simulink model "Robotic_Arm_For_SIMScape_2"  (R2020a)
settings: Solver=FixedStepAuto  StartTime=0.0  StopTime=70  FixedStep=0.01  RelTol=1e-3
model workspace: external: MATLAB File D:\jsp\Nottingham\Year 4\Semester 2\Third Year Project - Autonomous Robotic Arm\Software Development\SimScape\Version2\Robotic_Arm_For_SIMScape_2_DataFile.m (data not in the file)
values from neighbouring files (symbols this model uses):
  fcn11 = VariableA1(1)    [MainCode_16522575.m]
  fcn12 = VariableA1(2)    [MainCode_16522575.m]
  fcn13 = VariableA1(3)    [MainCode_16522575.m]
  fcn14 = VariableA1(4)    [MainCode_16522575.m]
  fcn1_1place = VariableA1toPlace(1)    [MainCode_16522575.m]
  fcn1_1placetoPrevious = VariableA1toPlacetoPrevious(1)    [MainCode_16522575.m]
  fcn1_2place = VariableA1toPlace(2)    [MainCode_16522575.m]
  fcn1_2placetoPrevious = VariableA1toPlacetoPrevious(2)    [MainCode_16522575.m]
  fcn1_3place = VariableA1toPlace(3)    [MainCode_16522575.m]
  fcn1_3placetoPrevious = VariableA1toPlacetoPrevious(3)    [MainCode_16522575.m]
  fcn1_4place = VariableA1toPlace(4)    [MainCode_16522575.m]
  fcn1_4placetoPrevious = VariableA1toPlacetoPrevious(4)    [MainCode_16522575.m]
  fcn21 = VariableA2(1)    [MainCode_16522575.m]
  fcn21home = VariableA2home(1)    [MainCode_16522575.m]
  fcn22 = VariableA2(2)    [MainCode_16522575.m]
  fcn22home = VariableA2home(2)    [MainCode_16522575.m]
  fcn23 = VariableA2(3)    [MainCode_16522575.m]
  fcn23home = VariableA2home(3)    [MainCode_16522575.m]
  fcn24 = VariableA2(4)    [MainCode_16522575.m]
  fcn24home = VariableA2home(4)    [MainCode_16522575.m]
  fcn2_1place = VariableA2toPlace(1)    [MainCode_16522575.m]
  fcn2_1placetohome = VariableA2toPlacetohome(1)    [MainCode_16522575.m]
  fcn2_2place = VariableA2toPlace(2)    [MainCode_16522575.m]
  fcn2_2placetohome = VariableA2toPlacetohome(2)    [MainCode_16522575.m]
  fcn2_3place = VariableA2toPlace(3)    [MainCode_16522575.m]
  fcn2_3placetohome = VariableA2toPlacetohome(3)    [MainCode_16522575.m]
  fcn2_4place = VariableA2toPlace(4)    [MainCode_16522575.m]
  fcn2_4placetohome = VariableA2toPlacetohome(4)    [MainCode_16522575.m]
  fcn31 = VariableA3(1)    [MainCode_16522575.m]
  fcn31home = VariableA3home(1)    [MainCode_16522575.m]
  fcn32 = VariableA3(2)    [MainCode_16522575.m]
  fcn32home = VariableA3home(2)    [MainCode_16522575.m]
  fcn33 = VariableA3(3)    [MainCode_16522575.m]
  fcn33home = VariableA3home(3)    [MainCode_16522575.m]
  fcn34 = VariableA3(4)    [MainCode_16522575.m]
  fcn34home = VariableA3home(4)    [MainCode_16522575.m]
  fcn3_1place = VariableA3toPlace(1)    [MainCode_16522575.m]
  fcn3_1placetohome = VariableA3toPlacetohome(1)    [MainCode_16522575.m]
  fcn3_2place = VariableA3toPlace(2)    [MainCode_16522575.m]
  fcn3_2placetohome = VariableA3toPlacetohome(2)    [MainCode_16522575.m]
  fcn3_3place = VariableA3toPlace(3)    [MainCode_16522575.m]
  fcn3_3placetohome = VariableA3toPlacetohome(3)    [MainCode_16522575.m]
  fcn3_4place = VariableA3toPlace(4)    [MainCode_16522575.m]
  fcn3_4placetohome = VariableA3toPlacetohome(4)    [MainCode_16522575.m]
  qd1_final = qd1(1000)    [TrajectoryPlanning.m]
  qd1_finalplace = qd1toPlace(1000)    [TrajectoryPlanning1toPlace.m]
  qd2_finalhome = qd2home(1000)    [TrajectoryPlanning2tohome.m]
  qd2_finalplacetohome = qd2toPlacetohome(1000)    [TrajectoryPlanning2Placetohome.m]
  qd2_initial = qd2(1)    [TrajectoryPlanning2.m]
  qd3_finalhome = qd3home(1000)    [TrajectoryPlanning3tohome.m]
  qd3_finalplacetohome = qd3toPlacetohome(1000)    [TrajectoryPlanning3Placetohome.m]
  qd3_initial = qd3(1)    [TrajectoryPlanning3.m]
  s = z-d1    [InverseKinematics.m]
undefined symbols (not defined in the file or in its folder): sigbuilder_block, smiData, X, Y, Z
libraries: sm_lib x32, nesl_utility x15
(part 1 of 2)
settings Model: Creator=sp_ja  LastModifiedBy=sp_ja
settings OptimizationCC: BlockReduction=off  DefaultParameterBehavior=Inlined  BufferReuse=off

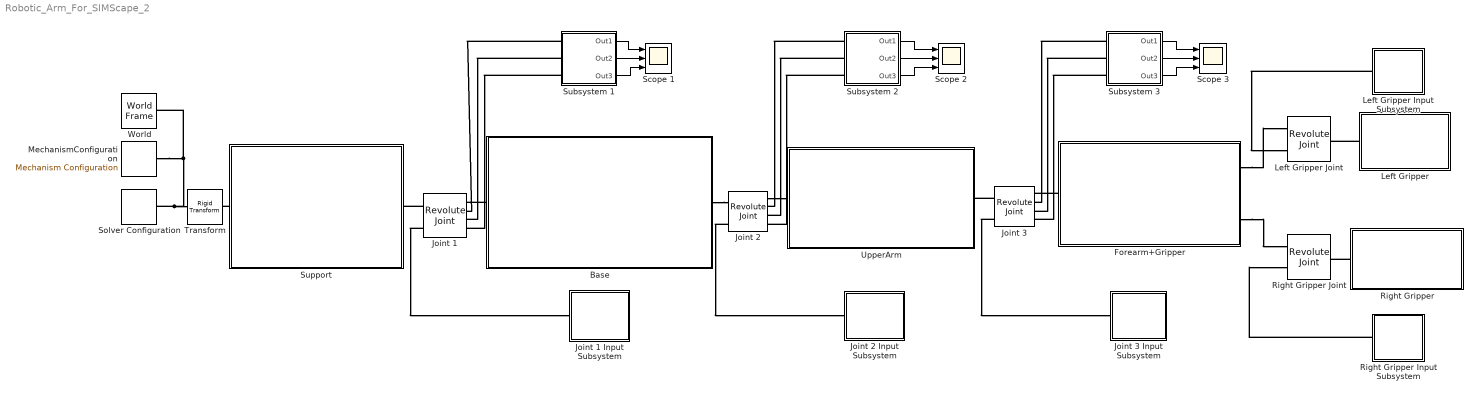
== system Robotic_Arm_For_SIMScape_2 ==
  Base : Subsystem
      mask Display: image('D:\jsp\Nottingham\Year 4\Semester 2\Third Year Project - Autonomous Robotic Arm\Software Development\SimScape\Version2\Pictures for Simulink\BaseNew.JPG'); % Use "Edit Image" on toolstrip to change.
  Forearm+Gripper : Subsystem
      mask Display: image('D:\jsp\Nottingham\Year 4\Semester 2\Third Year Project - Autonomous Robotic Arm\Software Development\SimScape\Version2\Pictures for Simulink\UpperArmNew3.JPG'); % Use "Edit Image" on toolstrip to change.
  "Joint 1 " : sm_lib/Joints/Revolute Joint  JointMode=Normal  SenseConstraintForce=off  SenseConstraintForceX=off  SenseConstraintForceY=off  SenseConstraintForceZ=off  SenseConstraintTorque=off  SenseConstraintTorqueX=off  SenseConstraintTorqueY=off  SenseConstraintTorqueZ=off  SenseTotalForce=off  SenseTotalForceX=off  SenseTotalForceY=off  SenseTotalForceZ=off  SenseTotalTorque=off  SenseTotalTorqueX=off  SenseTotalTorqueY=off  SenseTotalTorqueZ=off  CompositeWrenchDir=FollowerOnBase  CompositeWrenchFrame=BaseFrame  EquilibriumPosition=0  EquilibriumPositionUnits=rad  SpringStiffness=0  SpringStiffnessUnits=N*m/rad  DampingCoefficient=0  DampingCoefficientUnits=N*m/(rad/s)  TorqueActuationMode=ComputedTorque  MotionActuationMode=InputMotion  SensePosition=on  SenseVelocity=on  SenseAcceleration=on  SenseTorqueForce=off  SenseLowerLimitTorqueForce=off  SenseUpperLimitTorqueForce=off  LowerLimitSpecify=off  LowerLimitBound=-90  LowerLimitBoundUnits=deg  LowerLimitStiffness=1e4  LowerLimitStiffnessUnits=N*m/deg  LowerLimitDamping=10  LowerLimitDampingUnits=N*m/(deg/s)  LowerLimitTransitionRegionWidth=0.1  LowerLimitTransitionRegionWidthUnits=deg  UpperLimitSpecify=off  UpperLimitBound=90  UpperLimitBoundUnits=deg  UpperLimitStiffness=1e4  UpperLimitStiffnessUnits=N*m/deg  UpperLimitDamping=10  UpperLimitDampingUnits=N*m/(deg/s)  UpperLimitTransitionRegionWidth=0.1  UpperLimitTransitionRegionWidthUnits=deg  PositionTargetSpecify=on  PositionTargetPriority=Low  PositionTargetValue=smiData.RevoluteJoint(2).Rz.Pos  PositionTargetValueUnits=deg  VelocityTargetSpecify=off  VelocityTargetPriority=High  VelocityTargetValue=0  VelocityTargetValueUnits=deg/s
  Joint 1 Input Subsystem : Subsystem
      mask Display: image('D:\jsp\Nottingham\Year 4\Semester 2\Third Year Project - Autonomous Robotic Arm\Software Development\SimScape\Version2\Pictures for Simulink\return.png'); % Use "Edit Image" on toolstrip to change.
  Joint 2 : sm_lib/Joints/Revolute Joint  JointMode=Normal  SenseConstraintForce=off  SenseConstraintForceX=off  SenseConstraintForceY=off  SenseConstraintForceZ=off  SenseConstraintTorque=off  SenseConstraintTorqueX=off  SenseConstraintTorqueY=off  SenseConstraintTorqueZ=off  SenseTotalForce=off  SenseTotalForceX=off  SenseTotalForceY=off  SenseTotalForceZ=off  SenseTotalTorque=off  SenseTotalTorqueX=off  SenseTotalTorqueY=off  SenseTotalTorqueZ=off  CompositeWrenchDir=FollowerOnBase  CompositeWrenchFrame=BaseFrame  EquilibriumPosition=0  EquilibriumPositionUnits=rad  SpringStiffness=0  SpringStiffnessUnits=N*m/rad  DampingCoefficient=0  DampingCoefficientUnits=N*m/(rad/s)  TorqueActuationMode=ComputedTorque  MotionActuationMode=InputMotion  SensePosition=on  SenseVelocity=on  SenseAcceleration=on  SenseTorqueForce=off  SenseLowerLimitTorqueForce=off  SenseUpperLimitTorqueForce=off  LowerLimitSpecify=off  LowerLimitBound=-90  LowerLimitBoundUnits=deg  LowerLimitStiffness=1e4  LowerLimitStiffnessUnits=N*m/deg  LowerLimitDamping=10  LowerLimitDampingUnits=N*m/(deg/s)  LowerLimitTransitionRegionWidth=0.1  LowerLimitTransitionRegionWidthUnits=deg  UpperLimitSpecify=off  UpperLimitBound=90  UpperLimitBoundUnits=deg  UpperLimitStiffness=1e4  UpperLimitStiffnessUnits=N*m/deg  UpperLimitDamping=10  UpperLimitDampingUnits=N*m/(deg/s)  UpperLimitTransitionRegionWidth=0.1  UpperLimitTransitionRegionWidthUnits=deg  PositionTargetSpecify=on  PositionTargetPriority=Low  PositionTargetValue=smiData.RevoluteJoint(3).Rz.Pos  PositionTargetValueUnits=deg  VelocityTargetSpecify=off  VelocityTargetPriority=High  VelocityTargetValue=0  VelocityTargetValueUnits=deg/s
  Joint 2 Input Subsystem : Subsystem
      mask Display: image('D:\jsp\Nottingham\Year 4\Semester 2\Third Year Project - Autonomous Robotic Arm\Software Development\SimScape\Version2\Pictures for Simulink\return.png'); % Use "Edit Image" on toolstrip to change.
  Joint 3 : sm_lib/Joints/Revolute Joint  JointMode=Normal  SenseConstraintForce=off  SenseConstraintForceX=off  SenseConstraintForceY=off  SenseConstraintForceZ=off  SenseConstraintTorque=off  SenseConstraintTorqueX=off  SenseConstraintTorqueY=off  SenseConstraintTorqueZ=off  SenseTotalForce=off  SenseTotalForceX=off  SenseTotalForceY=off  SenseTotalForceZ=off  SenseTotalTorque=off  SenseTotalTorqueX=off  SenseTotalTorqueY=off  SenseTotalTorqueZ=off  CompositeWrenchDir=FollowerOnBase  CompositeWrenchFrame=BaseFrame  EquilibriumPosition=0  EquilibriumPositionUnits=rad  SpringStiffness=0  SpringStiffnessUnits=N*m/rad  DampingCoefficient=0  DampingCoefficientUnits=N*m/(rad/s)  TorqueActuationMode=ComputedTorque  MotionActuationMode=InputMotion  SensePosition=on  SenseVelocity=on  SenseAcceleration=on  SenseTorqueForce=off  SenseLowerLimitTorqueForce=off  SenseUpperLimitTorqueForce=off  LowerLimitSpecify=off  LowerLimitBound=-90  LowerLimitBoundUnits=deg  LowerLimitStiffness=1e4  LowerLimitStiffnessUnits=N*m/deg  LowerLimitDamping=10  LowerLimitDampingUnits=N*m/(deg/s)  LowerLimitTransitionRegionWidth=0.1  LowerLimitTransitionRegionWidthUnits=deg  UpperLimitSpecify=off  UpperLimitBound=90  UpperLimitBoundUnits=deg  UpperLimitStiffness=1e4  UpperLimitStiffnessUnits=N*m/deg  UpperLimitDamping=10  UpperLimitDampingUnits=N*m/(deg/s)  UpperLimitTransitionRegionWidth=0.1  UpperLimitTransitionRegionWidthUnits=deg  PositionTargetSpecify=on  PositionTargetPriority=Low  PositionTargetValue=smiData.RevoluteJoint(5).Rz.Pos  PositionTargetValueUnits=deg  VelocityTargetSpecify=off  VelocityTargetPriority=High  VelocityTargetValue=0  VelocityTargetValueUnits=deg/s
  Joint 3 Input Subsystem : Subsystem
      mask Display: image('D:\jsp\Nottingham\Year 4\Semester 2\Third Year Project - Autonomous Robotic Arm\Software Development\SimScape\Version2\Pictures for Simulink\return.png'); % Use "Edit Image" on toolstrip to change.
  Left Gripper : Subsystem
      mask Display: image('D:\jsp\Nottingham\Year 4\Semester 2\Third Year Project - Autonomous Robotic Arm\Software Development\SimScape\Version2\Pictures for Simulink\Gripper.JPG'); % Use "Edit Image" on toolstrip to change.
  Left Gripper Input Subsystem : Subsystem
      mask Display: image('D:\jsp\Nottingham\Year 4\Semester 2\Third Year Project - Autonomous Robotic Arm\Software Development\SimScape\Version2\Pictures for Simulink\return.png'); % Use "Edit Image" on toolstrip to change.
  Left Gripper Joint : sm_lib/Joints/Revolute Joint  JointMode=Normal  SenseConstraintForce=off  SenseConstraintForceX=off  SenseConstraintForceY=off  SenseConstraintForceZ=off  SenseConstraintTorque=off  SenseConstraintTorqueX=off  SenseConstraintTorqueY=off  SenseConstraintTorqueZ=off  SenseTotalForce=off  SenseTotalForceX=off  SenseTotalForceY=off  SenseTotalForceZ=off  SenseTotalTorque=off  SenseTotalTorqueX=off  SenseTotalTorqueY=off  SenseTotalTorqueZ=off  CompositeWrenchDir=FollowerOnBase  CompositeWrenchFrame=BaseFrame  EquilibriumPosition=0  EquilibriumPositionUnits=rad  SpringStiffness=0  SpringStiffnessUnits=N*m/rad  DampingCoefficient=0  DampingCoefficientUnits=N*m/(rad/s)  TorqueActuationMode=ComputedTorque  MotionActuationMode=InputMotion  SensePosition=off  SenseVelocity=off  SenseAcceleration=off  SenseTorqueForce=off  SenseLowerLimitTorqueForce=off  SenseUpperLimitTorqueForce=off  LowerLimitSpecify=off  LowerLimitBound=-90  LowerLimitBoundUnits=deg  LowerLimitStiffness=1e4  LowerLimitStiffnessUnits=N*m/deg  LowerLimitDamping=10  LowerLimitDampingUnits=N*m/(deg/s)  LowerLimitTransitionRegionWidth=0.1  LowerLimitTransitionRegionWidthUnits=deg  UpperLimitSpecify=off  UpperLimitBound=90  UpperLimitBoundUnits=deg  UpperLimitStiffness=1e4  UpperLimitStiffnessUnits=N*m/deg  UpperLimitDamping=10  UpperLimitDampingUnits=N*m/(deg/s)  UpperLimitTransitionRegionWidth=0.1  UpperLimitTransitionRegionWidthUnits=deg  PositionTargetSpecify=on  PositionTargetPriority=Low  PositionTargetValue=smiData.RevoluteJoint(4).Rz.Pos  PositionTargetValueUnits=deg  VelocityTargetSpecify=off  VelocityTargetPriority=High  VelocityTargetValue=0  VelocityTargetValueUnits=deg/s
  MechanismConfiguration : sm_lib/Utilities/Mechanism Configuration  UniformGravity=Constant  GravityVector=[0 -9.80665 0]  GravityUnits=m/s^2  LinearizationDelta=0.001
  Right Gripper : Subsystem
      mask Display: image('D:\jsp\Nottingham\Year 4\Semester 2\Third Year Project - Autonomous Robotic Arm\Software Development\SimScape\Version2\Pictures for Simulink\Gripper_with_Trigger.JPG'); % Use "Edit Image" on toolstrip to change.
  Right Gripper Input Subsystem : Subsystem
      mask Display: image('D:\jsp\Nottingham\Year 4\Semester 2\Third Year Project - Autonomous Robotic Arm\Software Development\SimScape\Version2\Pictures for Simulink\return.png'); % Use "Edit Image" on toolstrip to change.
  Right Gripper Joint : sm_lib/Joints/Revolute Joint  JointMode=Normal  SenseConstraintForce=off  SenseConstraintForceX=off  SenseConstraintForceY=off  SenseConstraintForceZ=off  SenseConstraintTorque=off  SenseConstraintTorqueX=off  SenseConstraintTorqueY=off  SenseConstraintTorqueZ=off  SenseTotalForce=off  SenseTotalForceX=off  SenseTotalForceY=off  SenseTotalForceZ=off  SenseTotalTorque=off  SenseTotalTorqueX=off  SenseTotalTorqueY=off  SenseTotalTorqueZ=off  CompositeWrenchDir=FollowerOnBase  CompositeWrenchFrame=BaseFrame  EquilibriumPosition=0  EquilibriumPositionUnits=rad  SpringStiffness=0  SpringStiffnessUnits=N*m/rad  DampingCoefficient=0  DampingCoefficientUnits=N*m/(rad/s)  TorqueActuationMode=ComputedTorque  MotionActuationMode=InputMotion  SensePosition=off  SenseVelocity=off  SenseAcceleration=off  SenseTorqueForce=off  SenseLowerLimitTorqueForce=off  SenseUpperLimitTorqueForce=off  LowerLimitSpecify=off  LowerLimitBound=-90  LowerLimitBoundUnits=deg  LowerLimitStiffness=1e4  LowerLimitStiffnessUnits=N*m/deg  LowerLimitDamping=10  LowerLimitDampingUnits=N*m/(deg/s)  LowerLimitTransitionRegionWidth=0.1  LowerLimitTransitionRegionWidthUnits=deg  UpperLimitSpecify=off  UpperLimitBound=90  UpperLimitBoundUnits=deg  UpperLimitStiffness=1e4  UpperLimitStiffnessUnits=N*m/deg  UpperLimitDamping=10  UpperLimitDampingUnits=N*m/(deg/s)  UpperLimitTransitionRegionWidth=0.1  UpperLimitTransitionRegionWidthUnits=deg  PositionTargetSpecify=on  PositionTargetPriority=Low  PositionTargetValue=smiData.RevoluteJoint(1).Rz.Pos  PositionTargetValueUnits=deg  VelocityTargetSpecify=off  VelocityTargetPriority=High  VelocityTargetValue=0  VelocityTargetValueUnits=deg/s
  Scope 1 : Scope  NumInputPorts=3
  Scope 2 : Scope  NumInputPorts=3
  Scope 3 : Scope  NumInputPorts=3
  Solver Configuration : nesl_utility/Solver Configuration  PhysicalDomain=network_engine_domain  SubClassName=solver  LeftPortType=input  RightPortType=generic  Tones=[]  Harmonics=[]  SimulateNoise=off  Profile=off  UseLocalSampling=off  EnableSwitchedLinearOptims=on  FrequencyDomain=off  UseCCode=off  RelTol=0.001  AbsTol=1e-06  MinStep=1e-09  ToWorkspace=off  RevertToSquareIcSolve=off  NumHomotopyIterations=100  PhasorMode=off  PhasorModeNumHarmonics=1  DoDC=off  ResidualTolerance=1e-09  UseLocalSolver=off  LocalSolverChoice=NE_BACKWARD_EULER_ADVANCER  LocalSolverSampleTime=0.001  DoFixedCost=off  MaxNonlinIter=3  MaxModeIter=2  LinearAlgebra=auto  EquationFormulation=NE_TIME_EF  DelaysMemoryBudget=1024  AutomaticFiltering=on  FilteringTimeConstant=0.001  PartitionStorageMethod=AS_NEEDED  PartitionMemoryBudget=1024  PartitionMethod=ROBUST
  Subsystem 1 : Subsystem
      mask Display: image('D:\jsp\Nottingham\Year 4\Semester 2\Third Year Project - Autonomous Robotic Arm\Software Development\SimScape\Version2\Pictures for Simulink\point-to.png'); % Use "Edit Image" on toolstrip to change.
  Subsystem 2 : Subsystem
      mask Display: image('D:\jsp\Nottingham\Year 4\Semester 2\Third Year Project - Autonomous Robotic Arm\Software Development\SimScape\Version2\Pictures for Simulink\point-to.png'); % Use "Edit Image" on toolstrip to change.
  Subsystem 3 : Subsystem
      mask Display: image('D:\jsp\Nottingham\Year 4\Semester 2\Third Year Project - Autonomous Robotic Arm\Software Development\SimScape\Version2\Pictures for Simulink\point-to.png'); % Use "Edit Image" on toolstrip to change.
  Support : Subsystem
      mask Display: image('D:\jsp\Nottingham\Year 4\Semester 2\Third Year Project - Autonomous Robotic Arm\Software Development\SimScape\Version2\Pictures for Simulink\SupportNew.JPG'); % Use "Edit Image" on toolstrip to change.
  Transform : sm_lib/Frames and Transforms/Rigid Transform  TranslationMethod=Cartesian  TranslationStandardOffset=0  TranslationLengthUnit=mm  TranslationStandardAxis=+Z  TranslationCartesianOffset=smiData.RigidTransform(12).translation  TranslationROffset=0  TranslationROffsetUnits=m  TranslationZOffset=0  TranslationZOffsetUnits=m  TranslationThetaOffset=0  TranslationThetaOffsetUnits=deg  RotationMethod=ArbitraryAxis  RotationAngleUnits=rad  RotationStandardAxis=+Z  RotationAngle=smiData.RigidTransform(12).angle  RotationArbitraryAxis=smiData.RigidTransform(12).axis  FollAlignAxisA=+X  BaseAlignAxisA=+Y  FollAlignAxisB=+Y  BaseAlignAxisB=+Z  RotationSequenceAxes=FollowerAxes  RotationSequence=XYX  RotationSequenceAngles=[0 0 0]  RotationSequenceAnglesUnits=deg  RotationMatrix=[1 0 0; 0 1 0; 0 0 1]
  UpperArm : Subsystem
      mask Display: image('D:\jsp\Nottingham\Year 4\Semester 2\Third Year Project - Autonomous Robotic Arm\Software Development\SimScape\Version2\Pictures for Simulink\Forearm + Gripper without offset.JPG'); % Use "Edit Image" on toolstrip to change.
  World : sm_lib/Frames and Transforms/World Frame
  wires:
  Subsystem 1/1(Out1) -> Scope 1/1
  Subsystem 1/2(Out2) -> Scope 1/2
  Subsystem 1/3(Out3) -> Scope 1/3
  Subsystem 2/1(Out1) -> Scope 2/1
  Subsystem 2/2(Out2) -> Scope 2/2
  Subsystem 2/3(Out3) -> Scope 2/3
  Subsystem 3/1(Out1) -> Scope 3/1
  Subsystem 3/2(Out2) -> Scope 3/2
  Subsystem 3/3(Out3) -> Scope 3/3
  connections:
  MechanismConfiguration/RConn1 -- Solver Configuration/RConn1 -- Transform/LConn1 -- World/RConn1
  Forearm+Gripper/RConn2 -- Right Gripper Joint/LConn1
  Forearm+Gripper/LConn1 -- Joint 3/RConn1
  Support/LConn1 -- Transform/RConn1
  Right Gripper/LConn1 -- Right Gripper Joint/RConn1
  "Joint 1 "/LConn1 -- Support/RConn1
  Base/LConn1 -- "Joint 1 "/RConn1
  Base/RConn1 -- Joint 2/LConn1
  Joint 2/RConn1 -- UpperArm/LConn1
  Forearm+Gripper/RConn1 -- Left Gripper Joint/LConn1
  Left Gripper/LConn1 -- Left Gripper Joint/RConn1
  Joint 3/LConn1 -- UpperArm/RConn1
  Subsystem 1/LConn1 -- "Joint 1 "/RConn2
  Subsystem 1/LConn2 -- "Joint 1 "/RConn3
  Subsystem 1/LConn3 -- "Joint 1 "/RConn4
  Subsystem 2/LConn1 -- Joint 2/RConn2
  Subsystem 2/LConn2 -- Joint 2/RConn3
  Subsystem 2/LConn3 -- Joint 2/RConn4
  Subsystem 3/LConn1 -- Joint 3/RConn2
  Subsystem 3/LConn2 -- Joint 3/RConn3
  Subsystem 3/LConn3 -- Joint 3/RConn4
  "Joint 1 "/LConn2 -- Joint 1 Input Subsystem/RConn1
  Joint 2/LConn2 -- Joint 2 Input Subsystem/RConn1
  Joint 3/LConn2 -- Joint 3 Input Subsystem/RConn1
  Right Gripper Input Subsystem/RConn1 -- Right Gripper Joint/LConn2
  Left Gripper Input Subsystem/RConn1 -- Left Gripper Joint/LConn2

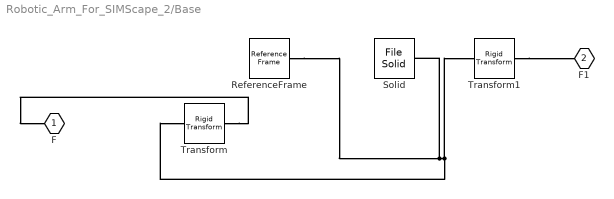
== system Robotic_Arm_For_SIMScape_2/Base ==
  ReferenceFrame : sm_lib/Frames and Transforms/Reference Frame
  Solid : sm_lib/Body Elements/File Solid  ExtGeomFileName=BaseNew_Default_sldprt.STEP  UnitType=FromFile  ExtGeomFileUnits=m  StepReaderType=HEX  ExportConvexHullGeometry=off  InertiaType=Custom  Mass=smiData.Solid(1).mass  MassUnits=kg  CenterOfMass=smiData.Solid(1).CoM  CenterOfMassUnits=mm  MomentsOfInertia=smiData.Solid(1).MoI  MomentsOfInertiaUnits=kg*mm^2  ProductsOfInertia=smiData.Solid(1).PoI  ProductsOfInertiaUnits=kg*mm^2  BasedOnType=DensityFromFile  Density=1000  DensityUnits=kg/m^3  DoExposeReferenceFrame=on  SerializedFrames=<Frames/>  GraphicType=FromGeometry  MarkerShape=Sphere  MarkerSize=10  GraphicVisPropType=AdvancedVisualProperties  GraphicDiffuseColor=[0.0 0.40392157 1.0]  GraphicSpecularColor=[0.5 0.5 0.5 1.0]  GraphicAmbientColor=[0.15 0.15 0.15 1.0]  GraphicEmissiveColor=[0.0 0.0 0.0 1.0]  GraphicShininess=10  GraphicOpacity=smiData.Solid(1).opacity
  Transform : sm_lib/Frames and Transforms/Rigid Transform  TranslationMethod=Cartesian  TranslationStandardOffset=0  TranslationLengthUnit=mm  TranslationStandardAxis=+Z  TranslationCartesianOffset=smiData.RigidTransform(4).translation  TranslationROffset=0  TranslationROffsetUnits=m  TranslationZOffset=0  TranslationZOffsetUnits=m  TranslationThetaOffset=0  TranslationThetaOffsetUnits=deg  RotationMethod=ArbitraryAxis  RotationAngleUnits=rad  RotationStandardAxis=+Z  RotationAngle=smiData.RigidTransform(4).angle  RotationArbitraryAxis=smiData.RigidTransform(4).axis  FollAlignAxisA=+X  BaseAlignAxisA=+Y  FollAlignAxisB=+Y  BaseAlignAxisB=+Z  RotationSequenceAxes=FollowerAxes  RotationSequence=XYX  RotationSequenceAngles=[0 0 0]  RotationSequenceAnglesUnits=deg  RotationMatrix=[1 0 0; 0 1 0; 0 0 1]
  Transform1 : sm_lib/Frames and Transforms/Rigid Transform  TranslationMethod=Cartesian  TranslationStandardOffset=0  TranslationLengthUnit=mm  TranslationStandardAxis=+Z  TranslationCartesianOffset=smiData.RigidTransform(5).translation  TranslationROffset=0  TranslationROffsetUnits=m  TranslationZOffset=0  TranslationZOffsetUnits=m  TranslationThetaOffset=0  TranslationThetaOffsetUnits=deg  RotationMethod=ArbitraryAxis  RotationAngleUnits=rad  RotationStandardAxis=+Z  RotationAngle=smiData.RigidTransform(5).angle  RotationArbitraryAxis=smiData.RigidTransform(5).axis  FollAlignAxisA=+Y  BaseAlignAxisA=+Z  FollAlignAxisB=+X  BaseAlignAxisB=+X  RotationSequenceAxes=BaseAxes  RotationSequence=XYZ  RotationSequenceAngles=[0 0 90]  RotationSequenceAnglesUnits=deg  RotationMatrix=[0 0 0; 0 0 0; 0 0 1]
  F : PMIOPort  Side=Left
  F1 : PMIOPort  Port=2  Side=Right
  connections:
  Solid/RConn1 -- ReferenceFrame/RConn1 -- Transform/LConn1 -- Transform1/LConn1
  Transform/RConn1 -- F/RConn1
  Transform1/RConn1 -- F1/RConn1

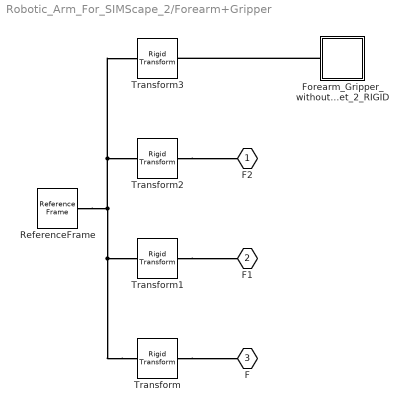
== system Robotic_Arm_For_SIMScape_2/Forearm+Gripper ==
  Forearm_Gripper_without_offset_2_RIGID : Subsystem
  ReferenceFrame : sm_lib/Frames and Transforms/Reference Frame
  Transform : sm_lib/Frames and Transforms/Rigid Transform  TranslationMethod=Cartesian  TranslationStandardOffset=0  TranslationLengthUnit=mm  TranslationStandardAxis=+Z  TranslationCartesianOffset=smiData.RigidTransform(1).translation  TranslationROffset=0  TranslationROffsetUnits=m  TranslationZOffset=0  TranslationZOffsetUnits=m  TranslationThetaOffset=0  TranslationThetaOffsetUnits=deg  RotationMethod=ArbitraryAxis  RotationAngleUnits=rad  RotationStandardAxis=+Z  RotationAngle=smiData.RigidTransform(1).angle  RotationArbitraryAxis=smiData.RigidTransform(1).axis  FollAlignAxisA=+X  BaseAlignAxisA=+Y  FollAlignAxisB=+Y  BaseAlignAxisB=+Z  RotationSequenceAxes=FollowerAxes  RotationSequence=XYX  RotationSequenceAngles=[0 0 0]  RotationSequenceAnglesUnits=deg  RotationMatrix=[1 0 0; 0 1 0; 0 0 1]
  Transform1 : sm_lib/Frames and Transforms/Rigid Transform  TranslationMethod=Cartesian  TranslationStandardOffset=0  TranslationLengthUnit=mm  TranslationStandardAxis=+Z  TranslationCartesianOffset=smiData.RigidTransform(7).translation  TranslationROffset=0  TranslationROffsetUnits=m  TranslationZOffset=0  TranslationZOffsetUnits=m  TranslationThetaOffset=0  TranslationThetaOffsetUnits=deg  RotationMethod=ArbitraryAxis  RotationAngleUnits=rad  RotationStandardAxis=+Z  RotationAngle=smiData.RigidTransform(7).angle  RotationArbitraryAxis=smiData.RigidTransform(7).axis  FollAlignAxisA=+X  BaseAlignAxisA=+Y  FollAlignAxisB=+Y  BaseAlignAxisB=+Z  RotationSequenceAxes=FollowerAxes  RotationSequence=XYX  RotationSequenceAngles=[0 0 0]  RotationSequenceAnglesUnits=deg  RotationMatrix=[1 0 0; 0 1 0; 0 0 1]
  Transform2 : sm_lib/Frames and Transforms/Rigid Transform  TranslationMethod=Cartesian  TranslationStandardOffset=0  TranslationLengthUnit=mm  TranslationStandardAxis=+Z  TranslationCartesianOffset=smiData.RigidTransform(10).translation  TranslationROffset=0  TranslationROffsetUnits=m  TranslationZOffset=0  TranslationZOffsetUnits=m  TranslationThetaOffset=0  TranslationThetaOffsetUnits=deg  RotationMethod=ArbitraryAxis  RotationAngleUnits=rad  RotationStandardAxis=+Z  RotationAngle=smiData.RigidTransform(10).angle  RotationArbitraryAxis=smiData.RigidTransform(10).axis  FollAlignAxisA=+X  BaseAlignAxisA=+Y  FollAlignAxisB=+Y  BaseAlignAxisB=+Z  RotationSequenceAxes=FollowerAxes  RotationSequence=XYX  RotationSequenceAngles=[0 0 0]  RotationSequenceAnglesUnits=deg  RotationMatrix=[1 0 0; 0 1 0; 0 0 1]
  Transform3 : sm_lib/Frames and Transforms/Rigid Transform  TranslationMethod=Cartesian  TranslationStandardOffset=0  TranslationLengthUnit=mm  TranslationStandardAxis=+Z  TranslationCartesianOffset=smiData.RigidTransform(11).translation  TranslationROffset=0  TranslationROffsetUnits=m  TranslationZOffset=0  TranslationZOffsetUnits=m  TranslationThetaOffset=0  TranslationThetaOffsetUnits=deg  RotationMethod=ArbitraryAxis  RotationAngleUnits=rad  RotationStandardAxis=+Z  RotationAngle=smiData.RigidTransform(11).angle  RotationArbitraryAxis=smiData.RigidTransform(11).axis  FollAlignAxisA=+X  BaseAlignAxisA=+Y  FollAlignAxisB=+Y  BaseAlignAxisB=+Z  RotationSequenceAxes=FollowerAxes  RotationSequence=XYX  RotationSequenceAngles=[0 0 0]  RotationSequenceAnglesUnits=deg  RotationMatrix=[1 0 0; 0 1 0; 0 0 1]
  F2 : PMIOPort  Side=Left
  F1 : PMIOPort  Port=2  Side=Right
  F : PMIOPort  Port=3  Side=Right
  connections:
  Transform/LConn1 -- ReferenceFrame/RConn1 -- Transform2/LConn1 -- Transform3/LConn1 -- Transform1/LConn1
  Transform/RConn1 -- F/RConn1
  Transform1/RConn1 -- F1/RConn1
  Transform2/RConn1 -- F2/RConn1
  Forearm_Gripper_without_offset_2_RIGID/LConn1 -- Transform3/RConn1

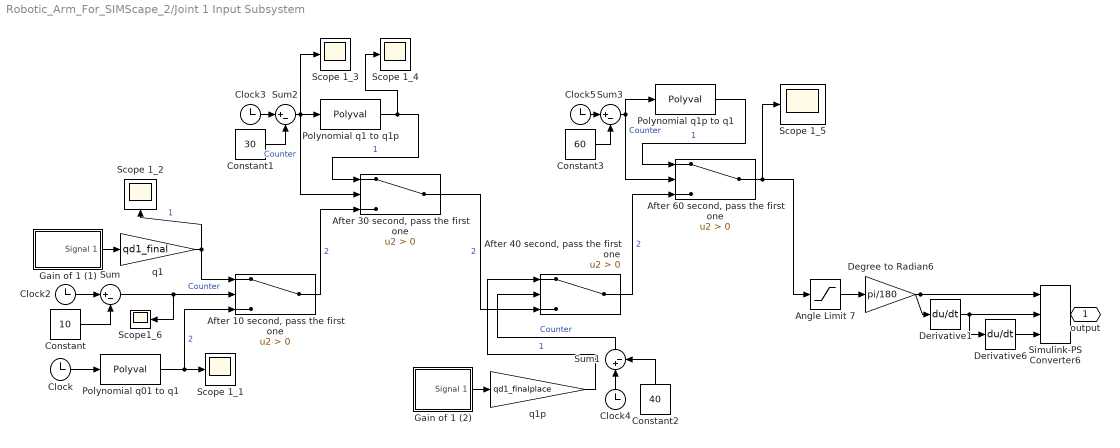
== system Robotic_Arm_For_SIMScape_2/Joint 1 Input Subsystem ==
  "After 10 second, pass the first one" : Switch  Criteria=u2 > Threshold
  "After 30 second, pass the first one" : Switch  Criteria=u2 > Threshold
  "After 40 second, pass the first one" : Switch  Criteria=u2 > Threshold
  "After 60 second, pass the first one" : Switch  Criteria=u2 > Threshold
  Angle Limit 7 : Saturate  UpperLimit=180  LowerLimit=-180
  Clock{,2..5} (5 alike) : Clock
      settings: Decimation=2000
      mask Display: image('C:\Users\sp_ja\Desktop\wall-clock.png'); % Use "Edit Image" on toolstrip to change.
  Constant : Constant  Value=10
  Constant1 : Constant  Value=30
  Constant2 : Constant  Value=40
  Constant3 : Constant  Value=60
  Degree to Radian6 : Gain  Gain=pi/180
  Derivative1 : Derivative  CoefficientInTFapproximation=1
  Derivative6 : Derivative  CoefficientInTFapproximation=1
  Gain of 1 (1) : Subsystem  Tag=STV Subsys  LoadFcn=sigbuilder_block('load');  StartFcn=sigbuilder_block('start');  StopFcn=sigbuilder_block('stop');  ClipboardFcn=sigbuilder_block('clipboard');  mask(Sigbuilder block){tuvar=[0:10]}
      mask help: Simulink:masks:SigbuilderBlock_MD
      mask init:
      | if ~strcmp(get_param(bdroot(gcbh),'SimulationStatus'),'stopped') tuvar = sigbuilder_block('maskInit'); end
      settings: CopyFcn=sigbuilder_block('copy');  DeleteFcn=sigbuilder_block('delete');  ModelCloseFcn=sigbuilder_block('modelClose');  PreSaveFcn=sigbuilder_block('preSave');  PauseFcn=sigbuilder_block('pause');  ContinueFcn=sigbuilder_block('continue');  NameChangeFcn=sigbuilder_block('namechange');  OpenFcn=sigbuilder_block('open',[437.6 199.2 550.4 400 ]);  CloseFcn=sigbuilder_block('close');
      mask Display: plot(0, 0, 100, 100,[2, 2, 32, 32, 2], [68, 8, 8, 68, 68],[32, 2], [38, 38], [32, 19, 2],[53, 60, 44], [32, 17, 17, 2],[16, 16, 31, 31]);txt = getActiveGroup(gcbh);text(2, 100, txt,'verticalAlignment', 'top');
  Gain of 1 (2) : Subsystem  Tag=STV Subsys  LoadFcn=sigbuilder_block('load');  StartFcn=sigbuilder_block('start');  StopFcn=sigbuilder_block('stop');  ClipboardFcn=sigbuilder_block('clipboard');  mask(Sigbuilder block){tuvar=[0:10]}
      mask help: Simulink:masks:SigbuilderBlock_MD
      mask init:
      | if ~strcmp(get_param(bdroot(gcbh),'SimulationStatus'),'stopped') tuvar = sigbuilder_block('maskInit'); end
      settings: CopyFcn=sigbuilder_block('copy');  DeleteFcn=sigbuilder_block('delete');  ModelCloseFcn=sigbuilder_block('modelClose');  PreSaveFcn=sigbuilder_block('preSave');  PauseFcn=sigbuilder_block('pause');  ContinueFcn=sigbuilder_block('continue');  NameChangeFcn=sigbuilder_block('namechange');  OpenFcn=sigbuilder_block('open',[448.2 144.6 550.8 400.2 ]);  CloseFcn=sigbuilder_block('close');
      mask Display: plot(0, 0, 100, 100,[2, 2, 32, 32, 2], [68, 8, 8, 68, 68],[32, 2], [38, 38], [32, 19, 2],[53, 60, 44], [32, 17, 17, 2],[16, 16, 31, 31]);txt = getActiveGroup(gcbh);text(2, 100, txt,'verticalAlignment', 'top');
  Polynomial q01 to q1 : Polyval  Coefs=[ fcn14 , fcn13 , fcn12 , fcn11]
  Polynomial q1 to q1p : Polyval  Coefs=[ fcn1_4place , fcn1_3place , fcn1_2place , fcn1_1place]
  Polynomial q1p to q1 : Polyval  Coefs=[ fcn1_4placetoPrevious , fcn1_3placetoPrevious , fcn1_2placetoPrevious , fcn1_1placetoPrevious]
  Scope 1_{1..5} (5 alike) : Scope
  Scope1_6 : Scope
  Simulink-PS Converter6 : nesl_utility/Simulink-PS Converter  PhysicalDomain=network_engine_domain  SubClassName=ps_input  LeftPortType=input  RightPortType=output  PseudoPeriodic=off  Frequencies=[]  NoiseDistribution=none  NoiseParameters=[]  Unit=1  AffineConversion=off  FilteringAndDerivatives=provide  SimscapeFilterOrder=1  InputFilterTimeConstant=0.001  UdotUserProvided=2
  Sum{,1..3} (4 alike) : Sum  Inputs=|+-
  q1 : Gain  Gain=qd1_final
  q1p : Gain  Gain=qd1_finalplace
  output : PMIOPort  Side=Right
  wires:
  Sum/1 -> "After 10 second, pass the first one"/2, Scope1_6/1  "Counter"
  Constant/1 -> Sum/2
  Clock2/1 -> Sum/1
  q1/1 -> "After 10 second, pass the first one"/1, Scope 1_2/1  "1"
  Gain of 1 (1)/1(Signal 1) -> q1/1
  Polynomial q01 to q1/1 -> "After 10 second, pass the first one"/3, Scope 1_1/1  "2"
  Clock/1 -> Polynomial q01 to q1/1
  "After 10 second, pass the first one"/1 -> "After 30 second, pass the first one"/3  "2"
  "After 30 second, pass the first one"/1 -> "After 40 second, pass the first one"/3  "2"
  Clock3/1 -> Sum2/1
  Constant1/1 -> Sum2/2
  Polynomial q1 to q1p/1 -> "After 30 second, pass the first one"/1, Scope 1_4/1  "1"
  Sum2/1 -> Scope 1_3/1, Polynomial q1 to q1p/1, "After 30 second, pass the first one"/2  "Counter"
  "After 40 second, pass the first one"/1 -> "After 60 second, pass the first one"/3  "2"
  Constant2/1 -> Sum1/2
  Clock4/1 -> Sum1/1
  Sum1/1 -> "After 40 second, pass the first one"/2  "Counter"
  Gain of 1 (2)/1(Signal 1) -> q1p/1
  q1p/1 -> "After 40 second, pass the first one"/1  "1"
  Sum3/1 -> "After 60 second, pass the first one"/2, Polynomial q1p to q1/1  "Counter"
  Clock5/1 -> Sum3/1
  Constant3/1 -> Sum3/2
  Derivative6/1 -> Simulink-PS Converter6/3
  Degree to Radian6/1 -> Derivative1/1, Simulink-PS Converter6/1
  Derivative1/1 -> Simulink-PS Converter6/2, Derivative6/1
  "After 60 second, pass the first one"/1 -> Angle Limit 7/1, Scope 1_5/1
  Angle Limit 7/1 -> Degree to Radian6/1
  Polynomial q1p to q1/1 -> "After 60 second, pass the first one"/1  "1"
  connections:
  output/RConn1 -- Simulink-PS Converter6/RConn1

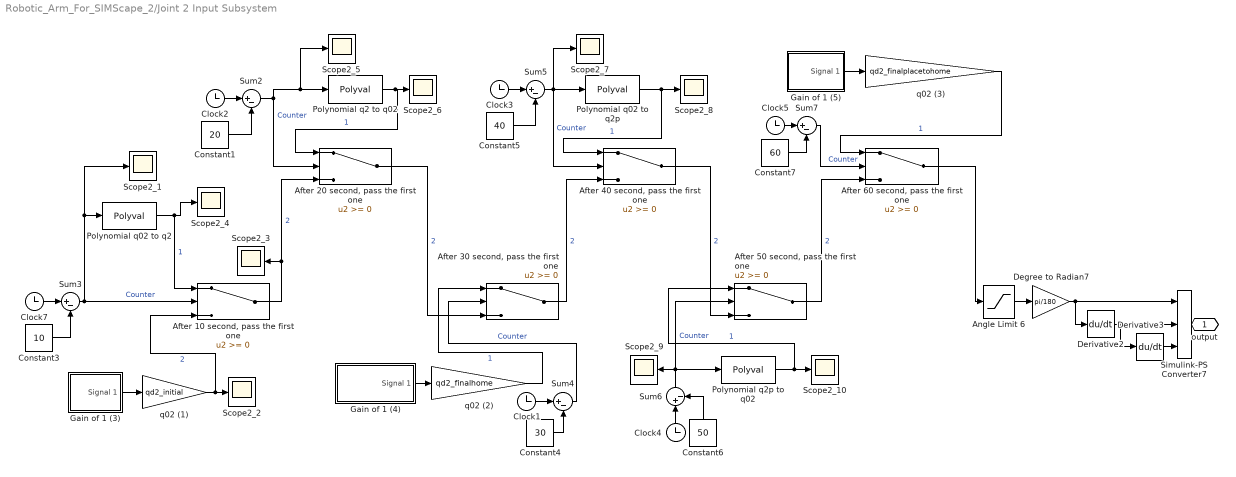
== system Robotic_Arm_For_SIMScape_2/Joint 2 Input Subsystem ==
  "After 10 second, pass the first one" : Switch
  "After 20 second, pass the first one" : Switch
  "After 30 second, pass the first one" : Switch
  "After 40 second, pass the first one" : Switch
  "After 50 second, pass the first one" : Switch
  "After 60 second, pass the first one" : Switch
  Angle Limit 6 : Saturate  UpperLimit=130  LowerLimit=0
  Clock{1..5,7} (6 alike) : Clock
      settings: Decimation=2000
      mask Display: image('C:\Users\sp_ja\Desktop\wall-clock.png'); % Use "Edit Image" on toolstrip to change.
  Constant1 : Constant  Value=20
  Constant3 : Constant  Value=10
  Constant4 : Constant  Value=30
  Constant5 : Constant  Value=40
  Constant6 : Constant  Value=50
  Constant7 : Constant  Value=60
  Degree to Radian7 : Gain  Gain=pi/180
  Derivative2 : Derivative  CoefficientInTFapproximation=1
  Derivative3 : Derivative  CoefficientInTFapproximation=1
  Gain of 1 (3) : Subsystem  Tag=STV Subsys  LoadFcn=sigbuilder_block('load');  StartFcn=sigbuilder_block('start');  StopFcn=sigbuilder_block('stop');  ClipboardFcn=sigbuilder_block('clipboard');  mask(Sigbuilder block){tuvar=[0:10]}
      mask help: Simulink:masks:SigbuilderBlock_MD
      mask init:
      | if ~strcmp(get_param(bdroot(gcbh),'SimulationStatus'),'stopped') tuvar = sigbuilder_block('maskInit'); end
      settings: CopyFcn=sigbuilder_block('copy');  DeleteFcn=sigbuilder_block('delete');  ModelCloseFcn=sigbuilder_block('modelClose');  PreSaveFcn=sigbuilder_block('preSave');  PauseFcn=sigbuilder_block('pause');  ContinueFcn=sigbuilder_block('continue');  NameChangeFcn=sigbuilder_block('namechange');  OpenFcn=sigbuilder_block('open',[437.6 199.2 550.4 400 ]);  CloseFcn=sigbuilder_block('close');
      mask Display: plot(0, 0, 100, 100,[2, 2, 32, 32, 2], [68, 8, 8, 68, 68],[32, 2], [38, 38], [32, 19, 2],[53, 60, 44], [32, 17, 17, 2],[16, 16, 31, 31]);txt = getActiveGroup(gcbh);text(2, 100, txt,'verticalAlignment', 'top');
  Gain of 1 (4) : Subsystem  Tag=STV Subsys  LoadFcn=sigbuilder_block('load');  StartFcn=sigbuilder_block('start');  StopFcn=sigbuilder_block('stop');  ClipboardFcn=sigbuilder_block('clipboard');  mask(Sigbuilder block){tuvar=[0:10]}
      mask help: Simulink:masks:SigbuilderBlock_MD
      mask init:
      | if ~strcmp(get_param(bdroot(gcbh),'SimulationStatus'),'stopped') tuvar = sigbuilder_block('maskInit'); end
      settings: CopyFcn=sigbuilder_block('copy');  DeleteFcn=sigbuilder_block('delete');  ModelCloseFcn=sigbuilder_block('modelClose');  PreSaveFcn=sigbuilder_block('preSave');  PauseFcn=sigbuilder_block('pause');  ContinueFcn=sigbuilder_block('continue');  NameChangeFcn=sigbuilder_block('namechange');  OpenFcn=sigbuilder_block('open',[437.6 199.2 550.4 400 ]);  CloseFcn=sigbuilder_block('close');
      mask Display: plot(0, 0, 100, 100,[2, 2, 32, 32, 2], [68, 8, 8, 68, 68],[32, 2], [38, 38], [32, 19, 2],[53, 60, 44], [32, 17, 17, 2],[16, 16, 31, 31]);txt = getActiveGroup(gcbh);text(2, 100, txt,'verticalAlignment', 'top');
  Gain of 1 (5) : Subsystem  Tag=STV Subsys  LoadFcn=sigbuilder_block('load');  StartFcn=sigbuilder_block('start');  StopFcn=sigbuilder_block('stop');  ClipboardFcn=sigbuilder_block('clipboard');  mask(Sigbuilder block){tuvar=[0:10]}
      mask help: Simulink:masks:SigbuilderBlock_MD
      mask init:
      | if ~strcmp(get_param(bdroot(gcbh),'SimulationStatus'),'stopped') tuvar = sigbuilder_block('maskInit'); end
      settings: CopyFcn=sigbuilder_block('copy');  DeleteFcn=sigbuilder_block('delete');  ModelCloseFcn=sigbuilder_block('modelClose');  PreSaveFcn=sigbuilder_block('preSave');  PauseFcn=sigbuilder_block('pause');  ContinueFcn=sigbuilder_block('continue');  NameChangeFcn=sigbuilder_block('namechange');  OpenFcn=sigbuilder_block('open',[437.6 199.2 550.4 400 ]);  CloseFcn=sigbuilder_block('close');
      mask Display: plot(0, 0, 100, 100,[2, 2, 32, 32, 2], [68, 8, 8, 68, 68],[32, 2], [38, 38], [32, 19, 2],[53, 60, 44], [32, 17, 17, 2],[16, 16, 31, 31]);txt = getActiveGroup(gcbh);text(2, 100, txt,'verticalAlignment', 'top');
  Polynomial q02 to q2 : Polyval  Coefs=[ fcn24 , fcn23 , fcn22 , fcn21]
  Polynomial q02 to q2p : Polyval  Coefs=[ fcn2_4place , fcn2_3place , fcn2_2place , fcn2_1place]
  Polynomial q2 to q02 : Polyval  Coefs=[ fcn24home , fcn23home , fcn22home , fcn21home]
  Polynomial q2p to q02 : Polyval  Coefs=[ fcn2_4placetohome , fcn2_3placetohome , fcn2_2placetohome , fcn2_1placetohome]
  Scope2_{1..10} (10 alike) : Scope
  Simulink-PS Converter7 : nesl_utility/Simulink-PS Converter  PhysicalDomain=network_engine_domain  SubClassName=ps_input  LeftPortType=input  RightPortType=output  PseudoPeriodic=off  Frequencies=[]  NoiseDistribution=none  NoiseParameters=[]  Unit=1  AffineConversion=off  FilteringAndDerivatives=provide  SimscapeFilterOrder=1  InputFilterTimeConstant=0.001  UdotUserProvided=2
  Sum{2..7} (6 alike) : Sum  Inputs=|+-
  q02 (1) : Gain  Gain=qd2_initial
  q02 (2) : Gain  Gain=qd2_finalhome
  q02 (3) : Gain  Gain=qd2_finalplacetohome
  output : PMIOPort  Side=Right
  wires:
  Polynomial q02 to q2/1 -> Scope2_4/1, "After 10 second, pass the first one"/1  "1"
  Gain of 1 (3)/1(Signal 1) -> q02 (1)/1
  Constant1/1 -> Sum2/2
  Clock2/1 -> Sum2/1
  "After 10 second, pass the first one"/1 -> "After 20 second, pass the first one"/3, Scope2_3/1  "2"
  Polynomial q2 to q02/1 -> "After 20 second, pass the first one"/1, Scope2_6/1  "1"
  Sum2/1 -> "After 20 second, pass the first one"/2, Scope2_5/1, Polynomial q2 to q02/1  "Counter"
  q02 (1)/1 -> Scope2_2/1, "After 10 second, pass the first one"/3  "2"
  Clock7/1 -> Sum3/1
  Constant3/1 -> Sum3/2
  Sum3/1 -> "After 10 second, pass the first one"/2, Polynomial q02 to q2/1, Scope2_1/1  "Counter"
  "After 20 second, pass the first one"/1 -> "After 30 second, pass the first one"/3  "2"
  Clock1/1 -> Sum4/1
  Constant4/1 -> Sum4/2
  Sum4/1 -> "After 30 second, pass the first one"/2  "Counter"
  Gain of 1 (4)/1(Signal 1) -> q02 (2)/1
  q02 (2)/1 -> "After 30 second, pass the first one"/1  "1"
  "After 30 second, pass the first one"/1 -> "After 40 second, pass the first one"/3  "2"
  Clock3/1 -> Sum5/1
  Constant5/1 -> Sum5/2
  Polynomial q02 to q2p/1 -> Scope2_8/1, "After 40 second, pass the first one"/1  "1"
  Sum5/1 -> Scope2_7/1, Polynomial q02 to q2p/1, "After 40 second, pass the first one"/2  "Counter"
  "After 50 second, pass the first one"/1 -> "After 60 second, pass the first one"/3  "2"
  "After 40 second, pass the first one"/1 -> "After 50 second, pass the first one"/3  "2"
  Constant6/1 -> Sum6/2
  Clock4/1 -> Sum6/1
  Sum6/1 -> Polynomial q2p to q02/1, "After 50 second, pass the first one"/2, Scope2_9/1  "Counter"
  Polynomial q2p to q02/1 -> Scope2_10/1, "After 50 second, pass the first one"/1  "1"
  Sum7/1 -> "After 60 second, pass the first one"/2  "Counter"
  Constant7/1 -> Sum7/2
  Clock5/1 -> Sum7/1
  q02 (3)/1 -> "After 60 second, pass the first one"/1  "1"
  Gain of 1 (5)/1(Signal 1) -> q02 (3)/1
  Degree to Radian7/1 -> Simulink-PS Converter7/1, Derivative2/1
  Derivative2/1 -> Simulink-PS Converter7/2, Derivative3/1
  Angle Limit 6/1 -> Degree to Radian7/1
  Derivative3/1 -> Simulink-PS Converter7/3
  "After 60 second, pass the first one"/1 -> Angle Limit 6/1
  connections:
  Simulink-PS Converter7/RConn1 -- output/RConn1

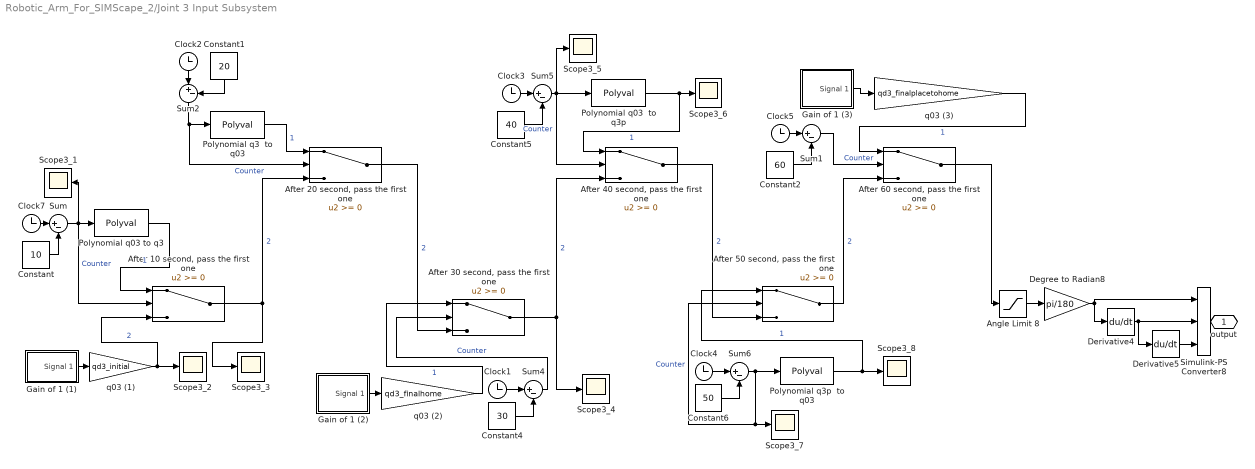
== system Robotic_Arm_For_SIMScape_2/Joint 3 Input Subsystem ==
  "After 10 second, pass the first one" : Switch
  "After 20 second, pass the first one" : Switch
  "After 30 second, pass the first one" : Switch
  "After 40 second, pass the first one" : Switch
  "After 50 second, pass the first one" : Switch
  "After 60 second, pass the first one" : Switch
  Angle Limit 8 : Saturate  UpperLimit=90  LowerLimit=-90
  Clock{1..5,7} (6 alike) : Clock
      settings: Decimation=2000
      mask Display: image('C:\Users\sp_ja\Desktop\wall-clock.png'); % Use "Edit Image" on toolstrip to change.
  Constant : Constant  Value=10
  Constant1 : Constant  Value=20
  Constant2 : Constant  Value=60
  Constant4 : Constant  Value=30
  Constant5 : Constant  Value=40
  Constant6 : Constant  Value=50
  Degree to Radian8 : Gain  Gain=pi/180
  Derivative4 : Derivative  CoefficientInTFapproximation=1
  Derivative5 : Derivative  CoefficientInTFapproximation=1
  Gain of 1 (1) : Subsystem  Tag=STV Subsys  LoadFcn=sigbuilder_block('load');  StartFcn=sigbuilder_block('start');  StopFcn=sigbuilder_block('stop');  ClipboardFcn=sigbuilder_block('clipboard');  mask(Sigbuilder block){tuvar=[0:10]}
      mask help: Simulink:masks:SigbuilderBlock_MD
      mask init:
      | if ~strcmp(get_param(bdroot(gcbh),'SimulationStatus'),'stopped') tuvar = sigbuilder_block('maskInit'); end
      settings: CopyFcn=sigbuilder_block('copy');  DeleteFcn=sigbuilder_block('delete');  ModelCloseFcn=sigbuilder_block('modelClose');  PreSaveFcn=sigbuilder_block('preSave');  PauseFcn=sigbuilder_block('pause');  ContinueFcn=sigbuilder_block('continue');  NameChangeFcn=sigbuilder_block('namechange');  OpenFcn=sigbuilder_block('open',[437.6 199.2 550.4 400 ]);  CloseFcn=sigbuilder_block('close');
      mask Display: plot(0, 0, 100, 100,[2, 2, 32, 32, 2], [68, 8, 8, 68, 68],[32, 2], [38, 38], [32, 19, 2],[53, 60, 44], [32, 17, 17, 2],[16, 16, 31, 31]);txt = getActiveGroup(gcbh);text(2, 100, txt,'verticalAlignment', 'top');
  Gain of 1 (2) : Subsystem  Tag=STV Subsys  LoadFcn=sigbuilder_block('load');  StartFcn=sigbuilder_block('start');  StopFcn=sigbuilder_block('stop');  ClipboardFcn=sigbuilder_block('clipboard');  mask(Sigbuilder block){tuvar=[0:10]}
      mask help: Simulink:masks:SigbuilderBlock_MD
      mask init:
      | if ~strcmp(get_param(bdroot(gcbh),'SimulationStatus'),'stopped') tuvar = sigbuilder_block('maskInit'); end
      settings: CopyFcn=sigbuilder_block('copy');  DeleteFcn=sigbuilder_block('delete');  ModelCloseFcn=sigbuilder_block('modelClose');  PreSaveFcn=sigbuilder_block('preSave');  PauseFcn=sigbuilder_block('pause');  ContinueFcn=sigbuilder_block('continue');  NameChangeFcn=sigbuilder_block('namechange');  OpenFcn=sigbuilder_block('open',[437.6 199.2 550.4 400 ]);  CloseFcn=sigbuilder_block('close');
      mask Display: plot(0, 0, 100, 100,[2, 2, 32, 32, 2], [68, 8, 8, 68, 68],[32, 2], [38, 38], [32, 19, 2],[53, 60, 44], [32, 17, 17, 2],[16, 16, 31, 31]);txt = getActiveGroup(gcbh);text(2, 100, txt,'verticalAlignment', 'top');
  Gain of 1 (3) : Subsystem  Tag=STV Subsys  LoadFcn=sigbuilder_block('load');  StartFcn=sigbuilder_block('start');  StopFcn=sigbuilder_block('stop');  ClipboardFcn=sigbuilder_block('clipboard');  mask(Sigbuilder block){tuvar=[0:10]}
      mask help: Simulink:masks:SigbuilderBlock_MD
      mask init:
      | if ~strcmp(get_param(bdroot(gcbh),'SimulationStatus'),'stopped') tuvar = sigbuilder_block('maskInit'); end
      settings: CopyFcn=sigbuilder_block('copy');  DeleteFcn=sigbuilder_block('delete');  ModelCloseFcn=sigbuilder_block('modelClose');  PreSaveFcn=sigbuilder_block('preSave');  PauseFcn=sigbuilder_block('pause');  ContinueFcn=sigbuilder_block('continue');  NameChangeFcn=sigbuilder_block('namechange');  OpenFcn=sigbuilder_block('open',[437.6 199.2 550.4 400 ]);  CloseFcn=sigbuilder_block('close');
      mask Display: plot(0, 0, 100, 100,[2, 2, 32, 32, 2], [68, 8, 8, 68, 68],[32, 2], [38, 38], [32, 19, 2],[53, 60, 44], [32, 17, 17, 2],[16, 16, 31, 31]);txt = getActiveGroup(gcbh);text(2, 100, txt,'verticalAlignment', 'top');
  Polynomial q03  to q3p : Polyval  Coefs=[ fcn3_4place , fcn3_3place , fcn3_2place , fcn3_1place]
  Polynomial q03 to q3 : Polyval  Coefs=[ fcn34 , fcn33 , fcn32 , fcn31]
  Polynomial q3  to q03 : Polyval  Coefs=[ fcn34home , fcn33home , fcn32home , fcn31home]
  Polynomial q3p  to q03 : Polyval  Coefs=[ fcn3_4placetohome , fcn3_3placetohome , fcn3_2placetohome , fcn3_1placetohome]
  Scope3_{1..8} (8 alike) : Scope
  Simulink-PS Converter8 : nesl_utility/Simulink-PS Converter  PhysicalDomain=network_engine_domain  SubClassName=ps_input  LeftPortType=input  RightPortType=output  PseudoPeriodic=off  Frequencies=[]  NoiseDistribution=none  NoiseParameters=[]  Unit=1  AffineConversion=off  FilteringAndDerivatives=provide  SimscapeFilterOrder=1  InputFilterTimeConstant=0.001  UdotUserProvided=2
  Sum{,1..2,4..6} (6 alike) : Sum  Inputs=|+-
  q03 (1) : Gain  Gain=qd3_initial
  q03 (2) : Gain  Gain=qd3_finalhome
  q03 (3) : Gain  Gain=qd3_finalplacetohome
  output : PMIOPort  Side=Right
  wires:
  Sum/1 -> "After 10 second, pass the first one"/2, Scope3_1/1, Polynomial q03 to q3/1  "Counter"
  Constant/1 -> Sum/2
  Clock7/1 -> Sum/1
  Polynomial q03 to q3/1 -> "After 10 second, pass the first one"/1  "1"
  q03 (1)/1 -> Scope3_2/1, "After 10 second, pass the first one"/3  "2"
  Gain of 1 (1)/1(Signal 1) -> q03 (1)/1
  "After 10 second, pass the first one"/1 -> Scope3_3/1, "After 20 second, pass the first one"/3  "2"
  Constant1/1 -> Sum2/2
  Clock2/1 -> Sum2/1
  Polynomial q3  to q03/1 -> "After 20 second, pass the first one"/1  "1"
  Sum2/1 -> Polynomial q3  to q03/1, "After 20 second, pass the first one"/2  "Counter"
  Constant4/1 -> Sum4/2
  Clock1/1 -> Sum4/1
  q03 (2)/1 -> "After 30 second, pass the first one"/1  "1"
  Sum4/1 -> "After 30 second, pass the first one"/2  "Counter"
  Gain of 1 (2)/1(Signal 1) -> q03 (2)/1
  "After 20 second, pass the first one"/1 -> "After 30 second, pass the first one"/3  "2"
  "After 30 second, pass the first one"/1 -> "After 40 second, pass the first one"/3, Scope3_4/1  "2"
  Sum5/1 -> Scope3_5/1, Polynomial q03  to q3p/1, "After 40 second, pass the first one"/2  "Counter"
  Constant5/1 -> Sum5/2
  Polynomial q03  to q3p/1 -> "After 40 second, pass the first one"/1, Scope3_6/1  "1"
  Clock3/1 -> Sum5/1
  Polynomial q3p  to q03/1 -> "After 50 second, pass the first one"/1, Scope3_8/1  "1"
  Clock4/1 -> Sum6/1
  Sum6/1 -> Polynomial q3p  to q03/1, "After 50 second, pass the first one"/2, Scope3_7/1  "Counter"
  "After 50 second, pass the first one"/1 -> "After 60 second, pass the first one"/3  "2"
  "After 40 second, pass the first one"/1 -> "After 50 second, pass the first one"/3  "2"
  Constant6/1 -> Sum6/2
  Gain of 1 (3)/1(Signal 1) -> q03 (3)/1
  q03 (3)/1 -> "After 60 second, pass the first one"/1  "1"
  Constant2/1 -> Sum1/2
  Clock5/1 -> Sum1/1
  Sum1/1 -> "After 60 second, pass the first one"/2  "Counter"
  Derivative4/1 -> Simulink-PS Converter8/2, Derivative5/1
  Degree to Radian8/1 -> Simulink-PS Converter8/1, Derivative4/1
  Derivative5/1 -> Simulink-PS Converter8/3
  Angle Limit 8/1 -> Degree to Radian8/1
  "After 60 second, pass the first one"/1 -> Angle Limit 8/1
  connections:
  Simulink-PS Converter8/RConn1 -- output/RConn1

== system Robotic_Arm_For_SIMScape_2/Left Gripper ==
  ReferenceFrame : sm_lib/Frames and Transforms/Reference Frame
  Solid : sm_lib/Body Elements/File Solid  ExtGeomFileName=Gripper_Default_sldprt.STEP  UnitType=FromFile  ExtGeomFileUnits=m  StepReaderType=HEX  ExportConvexHullGeometry=off  InertiaType=Custom  Mass=smiData.Solid(6).mass  MassUnits=kg  CenterOfMass=smiData.Solid(6).CoM  CenterOfMassUnits=mm  MomentsOfInertia=smiData.Solid(6).MoI  MomentsOfInertiaUnits=kg*mm^2  ProductsOfInertia=smiData.Solid(6).PoI  ProductsOfInertiaUnits=kg*mm^2  BasedOnType=DensityFromFile  Density=1000  DensityUnits=kg/m^3  DoExposeReferenceFrame=on  SerializedFrames=<Frames/>  GraphicType=FromGeometry  MarkerShape=Sphere  MarkerSize=10  GraphicVisPropType=AdvancedVisualProperties  GraphicDiffuseColor=smiData.Solid(6).color  GraphicSpecularColor=[0.5 0.5 0.5 1.0]  GraphicAmbientColor=[0.15 0.15 0.15 1.0]  GraphicEmissiveColor=[0.0 0.0 0.0 1.0]  GraphicShininess=1  GraphicOpacity=smiData.Solid(6).opacity
  Transform : sm_lib/Frames and Transforms/Rigid Transform  TranslationMethod=Cartesian  TranslationStandardOffset=0  TranslationLengthUnit=mm  TranslationStandardAxis=+Z  TranslationCartesianOffset=smiData.RigidTransform(8).translation  TranslationROffset=0  TranslationROffsetUnits=m  TranslationZOffset=0  TranslationZOffsetUnits=m  TranslationThetaOffset=0  TranslationThetaOffsetUnits=deg  RotationMethod=ArbitraryAxis  RotationAngleUnits=rad  RotationStandardAxis=+Z  RotationAngle=smiData.RigidTransform(8).angle  RotationArbitraryAxis=smiData.RigidTransform(8).axis  FollAlignAxisA=+X  BaseAlignAxisA=+Y  FollAlignAxisB=+Y  BaseAlignAxisB=+Z  RotationSequenceAxes=FollowerAxes  RotationSequence=XYX  RotationSequenceAngles=[0 0 0]  RotationSequenceAnglesUnits=deg  RotationMatrix=[1 0 0; 0 1 0; 0 0 1]
  F : PMIOPort  Side=Left
  connections:
  Solid/RConn1 -- ReferenceFrame/RConn1 -- Transform/LConn1
  Transform/RConn1 -- F/RConn1
